simulink model "LongitudinalTrim"  (R2020a)
settings: Solver=ode45  StartTime=0.0  StopTime=2  FixedStep=0.05  RelTol=1e-3
values from neighbouring files (symbols this model uses):
  data = cell2mat(rawdata)    [Mainbody.m]
  rawdata = datcomimport(path)    [Mainbody.m]
libraries: aerolibasang x5, aerolibadyn x2, aerolibconvert2 x1, aerolibatmos2 x1, shared3dof x1
settings Model: Creator=minec  LastModifiedBy=minec

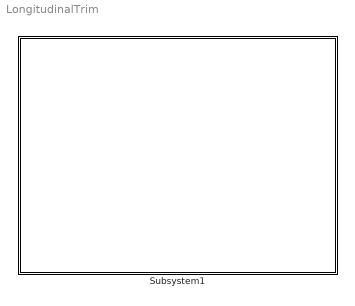
== system LongitudinalTrim ==
  Subsystem1 : Subsystem

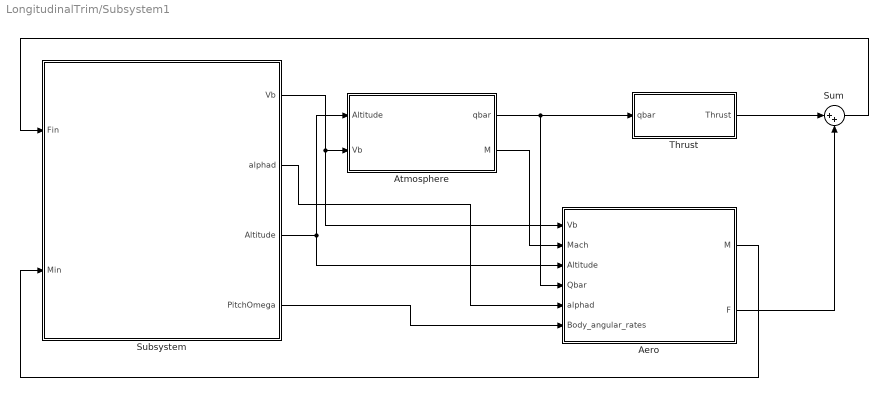
== system LongitudinalTrim/Subsystem1 ==
  Aero : Subsystem
  Atmosphere : Subsystem
  Subsystem : Subsystem
  Sum : Sum  Inputs=|++
  Thrust : Subsystem
  wires:
  Subsystem/1(Vb) -> Aero/1(Vb), Atmosphere/2(Vb)
  Atmosphere/1(qbar) -> Aero/4(Qbar), Thrust/1(qbar)
  Atmosphere/2(M) -> Aero/2(Mach)
  Subsystem/2(alphad) -> Aero/5(alphad)
  Subsystem/3(Altitude) -> Atmosphere/1(Altitude), Aero/3(Altitude)
  Subsystem/4(PitchOmega) -> Aero/6(Body_angular_rates)
  Sum/1 -> Subsystem/1(Fin)
  Aero/1(M) -> Subsystem/2(Min)
  Thrust/1(Thrust) -> Sum/1
  Aero/2(F) -> Sum/2

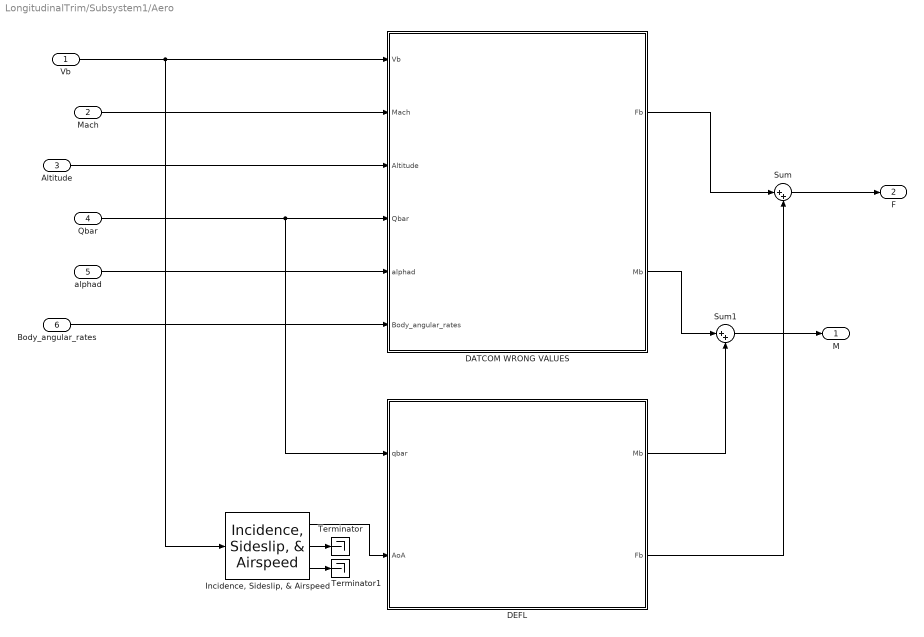
== system LongitudinalTrim/Subsystem1/Aero ==
  Vb : Inport
  Mach : Inport  Port=2
  Altitude : Inport  Port=3
  Qbar : Inport  Port=4
  alphad : Inport  Port=5
  Body_angular_rates : Inport  Port=6
  DATCOM WRONG VALUES : Subsystem
  DEFL : Subsystem
  "Incidence, Sideslip, & Airspeed" : aerolibasang/Incidence, Sideslip, & Airspeed
  Sum : Sum  Inputs=|++
  Sum1 : Sum  Inputs=|++
  Terminator : Terminator
  Terminator1 : Terminator
  M : Outport
  F : Outport  Port=2
  wires:
  Vb/1 -> "Incidence, Sideslip, & Airspeed"/1, DATCOM WRONG VALUES/1(Vb)
  Mach/1 -> DATCOM WRONG VALUES/2(Mach)
  Altitude/1 -> DATCOM WRONG VALUES/3(Altitude)
  Qbar/1 -> DEFL/1(qbar), DATCOM WRONG VALUES/4(Qbar)
  alphad/1 -> DATCOM WRONG VALUES/5(alphad)
  Body_angular_rates/1 -> DATCOM WRONG VALUES/6(Body_angular_rates)
  "Incidence, Sideslip, & Airspeed"/1 -> DEFL/2(AoA)
  "Incidence, Sideslip, & Airspeed"/2 -> Terminator/1
  "Incidence, Sideslip, & Airspeed"/3 -> Terminator1/1
  DATCOM WRONG VALUES/1(Fb) -> Sum/1
  DEFL/2(Fb) -> Sum/2
  DATCOM WRONG VALUES/2(Mb) -> Sum1/1
  DEFL/1(Mb) -> Sum1/2
  Sum1/1 -> M/1
  Sum/1 -> F/1

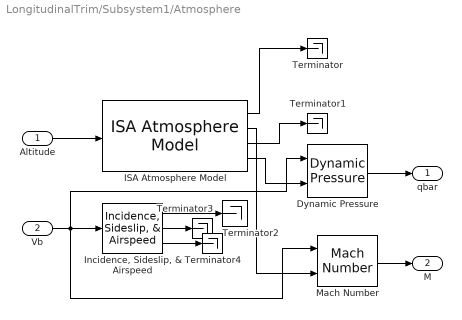
== system LongitudinalTrim/Subsystem1/Atmosphere ==
  Altitude : Inport
  Vb : Inport  Port=2
  Dynamic Pressure : aerolibasang/Dynamic Pressure
  ISA Atmosphere Model : aerolibatmos2/ISA Atmosphere Model  custom=off  g=9.80665  gamma=1.4  R=287.0531  L=0.0065  h_trop=11000  h_strat=20000  rho0=1.225  P0=101325  T0=288.15  h0=0
  "Incidence, Sideslip, & Airspeed" : aerolibasang/Incidence, Sideslip, & Airspeed
  Mach Number : aerolibasang/Mach Number
      settings: SourceProductBaseCode=AE
  Terminator{,1..4} (5 alike) : Terminator
  qbar : Outport
  M : Outport  Port=2
  wires:
  Altitude/1 -> ISA Atmosphere Model/1
  ISA Atmosphere Model/2 -> Mach Number/2
  ISA Atmosphere Model/3 -> Terminator1/1
  ISA Atmosphere Model/4 -> Dynamic Pressure/2
  ISA Atmosphere Model/1 -> Terminator/1
  "Incidence, Sideslip, & Airspeed"/1 -> Terminator2/1
  "Incidence, Sideslip, & Airspeed"/2 -> Terminator3/1
  Dynamic Pressure/1 -> qbar/1
  Vb/1 -> Mach Number/1, Dynamic Pressure/1, "Incidence, Sideslip, & Airspeed"/1
  Mach Number/1 -> M/1
  "Incidence, Sideslip, & Airspeed"/3 -> Terminator4/1

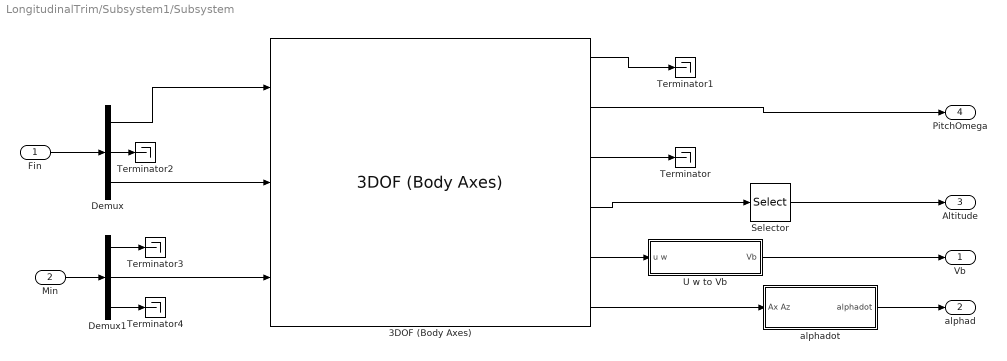
== system LongitudinalTrim/Subsystem1/Subsystem ==
  Fin : Inport
  Min : Inport  Port=2
  3DOF (Body Axes) : shared3dof/3DOF (Body Axes)  units=Metric (MKS)  mtype=Fixed  v_ini=140  theta_ini=0  alpha_ini=0  pos_ini=[0 3400]  q_ini=0  mass=data.mass  mass_e=0.5  mass_f=3.0  Iyy=data.inertia_yy  Iyy_e=0.5  Iyy_f=3.0  g_in=Internal  g=9.81  vre_flag=on  abi_flag=off  aMode=0  vel_statename=''  theta_statename=''  pos_statename=''  q_statename=''  mass_statename=''
      settings: SourceProductBaseCode=AE,PW,MT,VE,VP
  Demux : Demux  Outputs=3
  Demux1 : Demux  Outputs=3
  Selector : Selector  InputPortWidth=2  IndexOptions=Index vector (dialog)  Indices=[2]  OutputSizes=1
  Terminator{,1..4} (5 alike) : Terminator
  U w to Vb : Subsystem
  alphadot : Subsystem
  Vb : Outport
  alphad : Outport  Port=2
  Altitude : Outport  Port=3
  PitchOmega : Outport  Port=4
  wires:
  3DOF (Body Axes)/2 -> PitchOmega/1
  3DOF (Body Axes)/4 -> Selector/1
  3DOF (Body Axes)/5 -> U w to Vb/1(u w)
  3DOF (Body Axes)/6 -> alphadot/1(Ax Az)
  U w to Vb/1(Vb) -> Vb/1
  Selector/1 -> Altitude/1
  3DOF (Body Axes)/3 -> Terminator/1
  3DOF (Body Axes)/1 -> Terminator1/1
  Demux/2 -> Terminator2/1
  Demux/1 -> 3DOF (Body Axes)/1
  Demux/3 -> 3DOF (Body Axes)/2
  Fin/1 -> Demux/1
  Min/1 -> Demux1/1
  Demux1/2 -> 3DOF (Body Axes)/3
  Demux1/1 -> Terminator3/1
  Demux1/3 -> Terminator4/1
  alphadot/1(alphadot) -> alphad/1

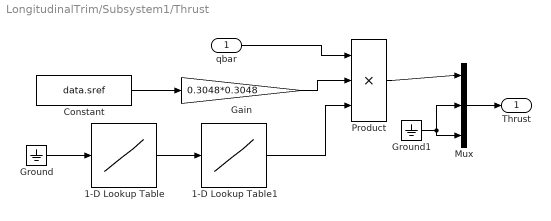
== system LongitudinalTrim/Subsystem1/Thrust ==
  qbar : Inport
  1-D Lookup Table : Lookup_n-D  NumberOfTableDimensions=1  BreakpointsForDimension1=-data.cm(~isnan(data.cm))  Table=data.alpha(~isnan(data.cm))  InternalRulePriority=Speed  RndMeth=Simplest  InputSameDT=on
  1-D Lookup Table1 : Lookup_n-D  NumberOfTableDimensions=1  BreakpointsForDimension1=data.alpha(~isnan(data.cd))  Table=data.cd(~isnan(data.cd))  InternalRulePriority=Speed  RndMeth=Simplest  InputSameDT=on
  Constant : Constant  Value=data.sref
  Gain : Gain  Gain=0.3048*0.3048
  Ground : Ground
  Ground1 : Ground
  Mux : Mux  Inputs=3
  Product : Product  Inputs=3
  Thrust : Outport
  wires:
  Ground/1 -> 1-D Lookup Table/1
  qbar/1 -> Product/1
  Product/1 -> Mux/1
  Mux/1 -> Thrust/1
  Ground1/1 -> Mux/2, Mux/3
  Gain/1 -> Product/2
  Constant/1 -> Gain/1
  1-D Lookup Table/1 -> 1-D Lookup Table1/1
  1-D Lookup Table1/1 -> Product/3

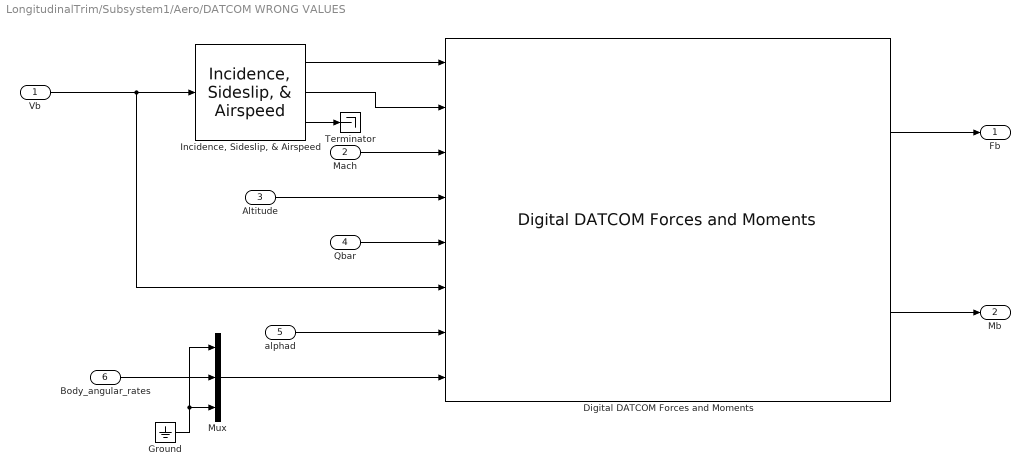
== system LongitudinalTrim/Subsystem1/Aero/DATCOM WRONG VALUES ==
  Vb : Inport
  Mach : Inport  Port=2
  Altitude : Inport  Port=3
  Qbar : Inport  Port=4
  alphad : Inport  Port=5
  Body_angular_rates : Inport  Port=6
  Digital DATCOM Forces and Moments : aerolibadyn/Digital DATCOM Forces and Moments  units=Metric (MKS)  dcase=rawdata{1}  fmode=Body  buildno=0  imethod=Linear  emethod=Linear  rmethod=Linear Extrapolation  action=None
      settings: SourceProductBaseCode=AE
  Ground : Ground
  "Incidence, Sideslip, & Airspeed" : aerolibasang/Incidence, Sideslip, & Airspeed
  Mux : Mux  Inputs=3
  Terminator : Terminator
  Fb : Outport
  Mb : Outport  Port=2
  wires:
  "Incidence, Sideslip, & Airspeed"/1 -> Digital DATCOM Forces and Moments/1
  alphad/1 -> Digital DATCOM Forces and Moments/7
  Qbar/1 -> Digital DATCOM Forces and Moments/5
  "Incidence, Sideslip, & Airspeed"/2 -> Digital DATCOM Forces and Moments/2
  Altitude/1 -> Digital DATCOM Forces and Moments/4
  Vb/1 -> "Incidence, Sideslip, & Airspeed"/1, Digital DATCOM Forces and Moments/6
  Digital DATCOM Forces and Moments/2 -> Mb/1
  Digital DATCOM Forces and Moments/1 -> Fb/1
  "Incidence, Sideslip, & Airspeed"/3 -> Terminator/1
  Mach/1 -> Digital DATCOM Forces and Moments/3
  Ground/1 -> Mux/1, Mux/3
  Mux/1 -> Digital DATCOM Forces and Moments/8
  Body_angular_rates/1 -> Mux/2

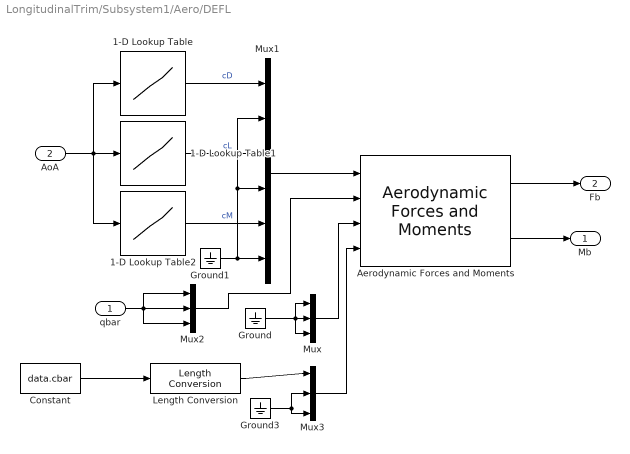
== system LongitudinalTrim/Subsystem1/Aero/DEFL ==
  qbar : Inport
  AoA : Inport  Port=2
  1-D Lookup Table : Lookup_n-D  NumberOfTableDimensions=1  BreakpointsForDimension1=data.alpha(~isnan(data.cd))  Table=data.cd(~isnan(data.cd))  InternalRulePriority=Speed  RndMeth=Simplest  InputSameDT=on
  1-D Lookup Table1 : Lookup_n-D  NumberOfTableDimensions=1  BreakpointsForDimension1=data.alpha(~isnan(data.cl))  Table=data.cl(~isnan(data.cl))  InternalRulePriority=Speed  RndMeth=Simplest  InputSameDT=on
  1-D Lookup Table2 : Lookup_n-D  NumberOfTableDimensions=1  BreakpointsForDimension1=data.alpha(~isnan(data.cm))  Table=data.cm(~isnan(data.cm))  InternalRulePriority=Speed  RndMeth=Simplest  InputSameDT=on
  "Aerodynamic Forces and Moments " : aerolibadyn/Aerodynamic Forces and Moments   inputAxes=Body  outputForceAxes=Body  outputMomentAxes=Body  S=data.sref*0.3048^2  b=data.blref*0.3048  cbar=data.cbar*0.3048
  Constant : Constant  Value=data.cbar
  Ground : Ground
  Ground1 : Ground
  Ground3 : Ground
  Length Conversion : aerolibconvert2/Length Conversion  IU=ft  OU=m
  Mux : Mux  Inputs=3
  Mux1 : Mux  Inputs=6
  Mux2 : Mux  Inputs=3
  Mux3 : Mux  Inputs=3
  Mb : Outport
  Fb : Outport  Port=2
  wires:
  Ground/1 -> Mux/3, Mux/1, Mux/2
  1-D Lookup Table/1 -> Mux1/1  "cD"
  AoA/1 -> 1-D Lookup Table2/1, 1-D Lookup Table1/1, 1-D Lookup Table/1
  1-D Lookup Table1/1 -> Mux1/3  "cL"
  1-D Lookup Table2/1 -> Mux1/5  "cM"
  Ground1/1 -> Mux1/2, Mux1/4, Mux1/6
  Mux1/1 -> "Aerodynamic Forces and Moments "/1
  "Aerodynamic Forces and Moments "/2 -> Mb/1
  Mux2/1 -> "Aerodynamic Forces and Moments "/2
  Ground3/1 -> Mux3/2, Mux3/3
  Mux/1 -> "Aerodynamic Forces and Moments "/3
  Mux3/1 -> "Aerodynamic Forces and Moments "/4
  qbar/1 -> Mux2/2, Mux2/3, Mux2/1
  Length Conversion/1 -> Mux3/1
  Constant/1 -> Length Conversion/1
  "Aerodynamic Forces and Moments "/1 -> Fb/1

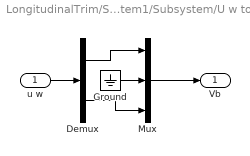
== system LongitudinalTrim/Subsystem1/Subsystem/U w to Vb ==
  u w : Inport
  Demux : Demux  Outputs=2
  Ground : Ground
  Mux : Mux  Inputs=3
  Vb : Outport
  wires:
  u w/1 -> Demux/1
  Ground/1 -> Mux/2
  Demux/1 -> Mux/1
  Demux/2 -> Mux/3
  Mux/1 -> Vb/1

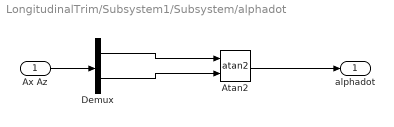
== system LongitudinalTrim/Subsystem1/Subsystem/alphadot ==
  Ax Az : Inport
  Atan2 : Trigonometry  Operator=atan2
  Demux : Demux  Outputs=2
  alphadot : Outport
  wires:
  Ax Az/1 -> Demux/1
  Demux/1 -> Atan2/1
  Demux/2 -> Atan2/2
  Atan2/1 -> alphadot/1
